simulink model "untitled1"  (R2020b)
settings: Solver=FixedStepDiscrete  StartTime=0.0  StopTime=10.0  FixedStep=200e-6  RelTol=1e-3
libraries: simulink x7
settings Model: PacingRate=100  Creator=unix  LastModifiedBy=unix

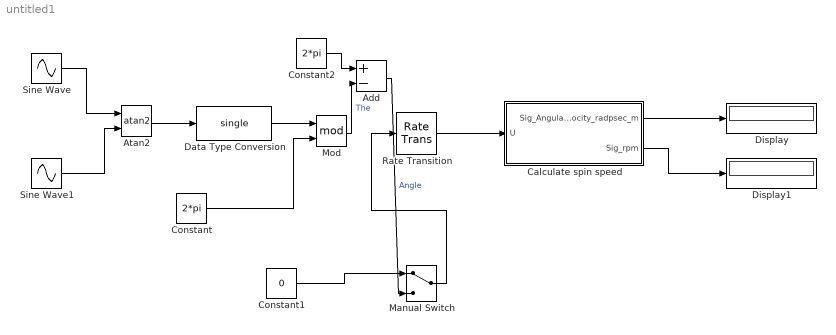
== system untitled1 ==
  Add : Sum  Inputs=+-
  Atan2 : Trigonometry  Operator=atan2
  Calculate spin speed : Subsystem  TreatAsAtomicUnit=on
  Constant : Constant  Value=2*pi  OutDataTypeStr=single
  Constant1 : Constant  Value=0  OutDataTypeStr=single
  Constant2 : Constant  Value=2*pi  OutDataTypeStr=Inherit: Inherit via back propagation
  Data Type Conversion : DataTypeConversion  OutDataTypeStr=single
  Display : Display
  Display1 : Display
  Manual Switch : ManualSwitch
  Mod : Math  Operator=mod  SaturateOnIntegerOverflow=on
  Rate Transition : RateTransition
  Sine Wave : Sin  Frequency=100  SampleTime=0
  Sine Wave1 : Sin  Frequency=100  Phase=pi/2  SampleTime=0
  wires:
  Sine Wave/1 -> Atan2/1
  Sine Wave1/1 -> Atan2/2
  Atan2/1 -> Data Type Conversion/1
  Data Type Conversion/1 -> Mod/1
  Constant/1 -> Mod/2
  Calculate spin speed/1(Sig_Angular_Velocity_radpsec_m) -> Display/1
  Calculate spin speed/2(Sig_rpm) -> Display1/1
  Rate Transition/1 -> Calculate spin speed/1(U)
  Constant2/1 -> Add/1
  Mod/1 -> Add/2  "The"
  Add/1 -> Manual Switch/2  "Angle"
  Constant1/1 -> Manual Switch/1
  Manual Switch/1 -> Rate Transition/1

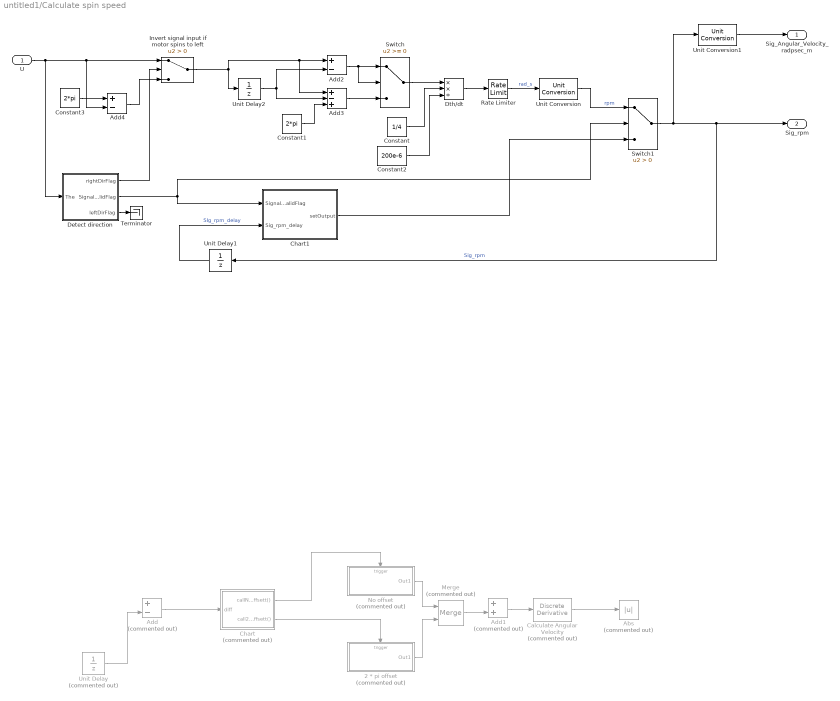
== system untitled1/Calculate spin speed ==
  U : Inport
  2 * pi offset : Subsystem  Commented=on  TreatAsAtomicUnit=on
  Abs : Abs  Commented=on
  Add : Sum  Commented=on  Inputs=+-
  Add1 : Sum  Commented=on
  Add2 : Sum  Inputs=+-
  Add3 : Sum  Inputs=+-+
  Add4 : Sum  Inputs=+-
  Calculate Angular Velocity : simulink/Discrete/Discrete Derivative  Commented=on  gainval=1.0  ICPrevScaledInput=0.0  OutMin=[]  OutMax=[]  OutDataTypeStr=single  OutputDataTypeScalingMode=single  OutDataType=fixdt(1, 16)  OutScaling=2^-10  DoSatur=off
  Chart : Stateflow chart  Commented=on  TreatAsAtomicUnit=on
  Chart1 : Stateflow chart  TreatAsAtomicUnit=on
  Constant : Constant  Value=1/4  OutDataTypeStr=single
  Constant1 : Constant  Value=2*pi  OutDataTypeStr=single
  Constant2 : Constant  Value=200e-6  OutDataTypeStr=single
  Constant3 : Constant  Value=2*pi  OutDataTypeStr=Inherit: Inherit via back propagation
  "Detect direction " : Subsystem
  Dth/dt : Product  Inputs=**/
  Invert signal input if motor spins to left : Switch  Criteria=u2 > Threshold
  Merge : Merge  Commented=on
  No offset : Subsystem  Commented=on  TreatAsAtomicUnit=on
  Rate Limiter : RateLimiter  RisingSlewLimit=50000  FallingSlewLimit=-50000  SampleTimeMode=inherited
  Switch : Switch  OutDataTypeStr=single
  Switch1 : Switch  Criteria=u2 > Threshold  OutDataTypeStr=single
  Terminator : Terminator
  Unit Conversion : UnitConversion
  Unit Conversion1 : UnitConversion  OutputType=Inherit: Inherit via back propagation
  Unit Delay : UnitDelay  Commented=on  SampleTime=-1  HasFrameUpgradeWarning=on
  Unit Delay1 : UnitDelay  SampleTime=-1  HasFrameUpgradeWarning=on
  Unit Delay2 : UnitDelay  SampleTime=-1  HasFrameUpgradeWarning=on
  Sig_Angular_Velocity_radpsec_m : Outport  Unit=rad/sec
  Sig_rpm : Outport  Port=2  Unit=rpm
  wires:
  Rate Limiter/1 -> Unit Conversion/1  "rad_s"
  Add3/1 -> Switch/3
  Unit Delay2/1 -> Add3/2, Add2/2
  Switch/1 -> Dth/dt/1
  Add2/1 -> Switch/2, Switch/1
  Constant1/1 -> Add3/3
  Chart/1(callNoOffsett()) -> No offset/Trigger
  No offset/1(Out1) -> Merge/1
  Calculate Angular Velocity/1 -> Abs/1
  Chart/2(call2PiOffsett()) -> 2 * pi offset/Trigger
  2 * pi offset/1(Out1) -> Merge/2
  Add1/1 -> Calculate Angular Velocity/1
  Add/1 -> Chart/1(diff)
  Merge/1 -> Add1/2
  Unit Delay/1 -> Add/2
  ? -> Unit Delay/1, Add1/1, Add/1
  Constant/1 -> Dth/dt/2
  "Detect direction "/1(rightDirFlag) -> Invert signal input if motor spins to left/2
  Constant3/1 -> Add4/1
  U/1 -> Add4/2, Invert signal input if motor spins to left/1, "Detect direction "/1(The)
  Add4/1 -> Invert signal input if motor spins to left/3
  Invert signal input if motor spins to left/1 -> Unit Delay2/1, Add3/1, Add2/1
  "Detect direction "/3(leftDirFlag) -> Terminator/1
  "Detect direction "/2(SignalValidFlag) -> Switch1/2, Chart1/1(SignalValidFlag)
  Unit Delay1/1 -> Chart1/2(Sig_rpm_delay)  "SIg_rpm_delay"
  Switch1/1 -> Unit Conversion1/1, Sig_rpm/1, Unit Delay1/1  "Sig_rpm"
  Chart1/1(setOutput) -> Switch1/3
  Unit Conversion/1 -> Switch1/1  "rpm"
  Unit Conversion1/1 -> Sig_Angular_Velocity_radpsec_m/1
  Constant2/1 -> Dth/dt/3
  Dth/dt/1 -> Rate Limiter/1

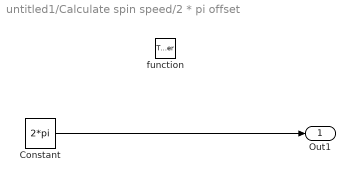
== system untitled1/Calculate spin speed/2 * pi offset ==
  function : TriggerPort  TriggerType=function-call  VariantControl=Variant
  Constant : Constant  Value=2*pi  OutDataTypeStr=single
  Out1 : Outport
  wires:
  Constant/1 -> Out1/1

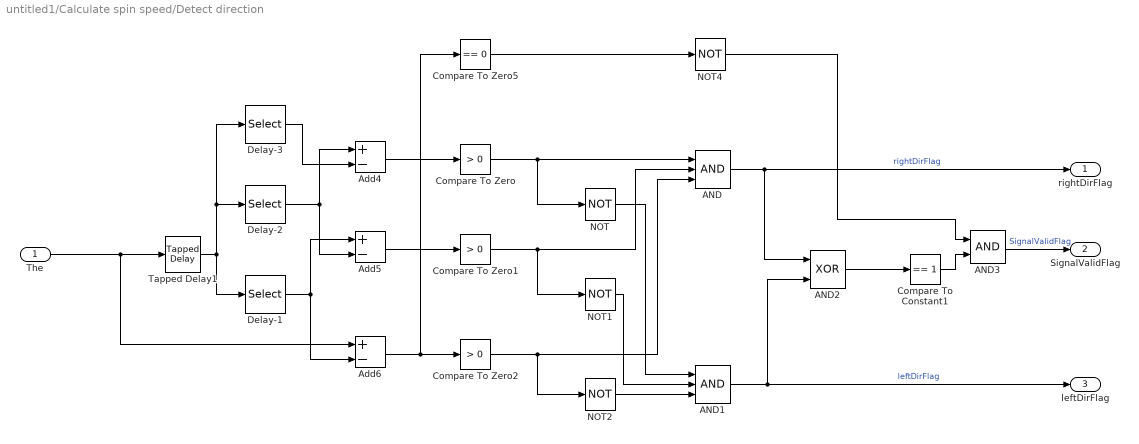
== system untitled1/Calculate spin speed/Detect direction  ==
  The : Inport
  AND : Logic  Inputs=3  AllPortsSameDT=off  OutDataTypeStr=boolean
  AND1 : Logic  Inputs=3  AllPortsSameDT=off  OutDataTypeStr=boolean
  AND2 : Logic  Operator=XOR  AllPortsSameDT=off  OutDataTypeStr=boolean
  AND3 : Logic  AllPortsSameDT=off  OutDataTypeStr=boolean
  Add4 : Sum  Inputs=+-
  Add5 : Sum  Inputs=+-
  Add6 : Sum  Inputs=+-
  Compare To Constant1 : simulink/Logic and Bit Operations/Compare To Constant  relop===  const=1  OutDataTypeStr=boolean
  Compare To Zero : simulink/Logic and Bit Operations/Compare To Zero  relop=>  OutDataTypeStr=boolean
  Compare To Zero1 : simulink/Logic and Bit Operations/Compare To Zero  relop=>  OutDataTypeStr=boolean
  Compare To Zero2 : simulink/Logic and Bit Operations/Compare To Zero  relop=>  OutDataTypeStr=boolean
  Compare To Zero5 : simulink/Logic and Bit Operations/Compare To Zero  relop===  OutDataTypeStr=boolean
  Delay-1 : Selector  InputPortWidth=3  IndexOptions=Index vector (dialog)  Indices=3  OutputSizes=1
  Delay-2 : Selector  InputPortWidth=3  IndexOptions=Index vector (dialog)  Indices=2  OutputSizes=1
  Delay-3 : Selector  InputPortWidth=3  IndexOptions=Index vector (dialog)  Indices=1  OutputSizes=1
  NOT{,1..2,4} (4 alike) : Logic  Operator=NOT  IconShape=distinctive  AllPortsSameDT=off  OutDataTypeStr=boolean
  Tapped Delay1 : simulink/Discrete/Tapped Delay  vinit=0.0  samptime=-1  NumDelays=3  DelayOrder=Oldest  includeCurrent=off
  rightDirFlag : Outport
  SignalValidFlag : Outport  Port=2
  leftDirFlag : Outport  Port=3
  wires:
  Add4/1 -> Compare To Zero/1
  Delay-1/1 -> Add5/1, Add6/2
  Delay-3/1 -> Add4/2
  Compare To Zero2/1 -> NOT2/1, AND/3
  NOT1/1 -> AND1/2
  Add6/1 -> Compare To Zero5/1, Compare To Zero2/1
  Add5/1 -> Compare To Zero1/1
  AND1/1 -> leftDirFlag/1, AND2/2  "leftDirFlag"
  AND/1 -> rightDirFlag/1, AND2/1  "rightDirFlag"
  Delay-2/1 -> Add4/1, Add5/2
  Compare To Zero/1 -> AND/1, NOT/1
  Tapped Delay1/1 -> Delay-1/1, Delay-2/1, Delay-3/1
  NOT/1 -> AND1/1
  NOT2/1 -> AND1/3
  The/1 -> Tapped Delay1/1, Add6/1
  Compare To Zero1/1 -> NOT1/1, AND/2
  AND3/1 -> SignalValidFlag/1  "SignalValidFlag"
  AND2/1 -> Compare To Constant1/1
  Compare To Zero5/1 -> NOT4/1
  NOT4/1 -> AND3/1
  Compare To Constant1/1 -> AND3/2

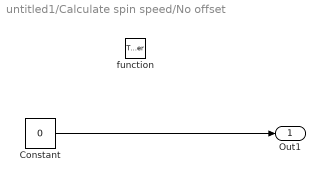
== system untitled1/Calculate spin speed/No offset ==
  function : TriggerPort  TriggerType=function-call  VariantControl=Variant
  Constant : Constant  Value=0  OutDataTypeStr=single
  Out1 : Outport
  wires:
  Constant/1 -> Out1/1

== stateflow chart untitled1/Calculate spin speed/Chart1 ==
  state InvalidSignal
    en:count = count + 1;
    state noTimeout
      du:count++;
      state MotorWasInRotation
        en:setOutput=Sig_rpm_delay;
        du:setOutput=Sig_rpm_delay;
      state MotorWasStalled
        en:setOutput=0;
        du:setOutput=0;
      (default) -> (junction 60)
      (junction 60) -> MotorWasStalled [order 2]
      (junction 60) -> MotorWasInRotation [order 1] : [Sig_rpm_delay!=0]
    state timeout
      en:setOutput=0;
    (default) -> noTimeout
    noTimeout -> timeout : [count>3]
  state ValidSignal1
    du:count = 0;
  (default) -> (junction 48)
  (junction 48) -> ValidSignal1 [order 2]
  (junction 48) -> InvalidSignal [order 1] : [SignalValidFlag==0]
  InvalidSignal -> ValidSignal1 : [SignalValidFlag==1]
  ValidSignal1 -> InvalidSignal : [SignalValidFlag==0]
  data: SignalValidFlag input; Sig_rpm_delay input; count local uint8; setOutput output double

== stateflow chart untitled1/Calculate spin speed/Chart ==
  (default) -> (junction 2)
  (junction 2) -> (junction 4) [order 1] : [diff<0]{call2PiOffsett()}
  (junction 2) -> (junction 6) [order 2] : [diff>=0]{callNoOffsett()}
  (junction 4) -> (junction 8)
  (junction 8) -> (junction 6)
  (junction 6) -> (junction 11)
  data: diff input
  events: callNoOffsett output FUNCTION_CALL_EVENT; call2PiOffsett output FUNCTION_CALL_EVENT
